simulink model "untitled"  (R2025a)
settings: Solver=VariableStepAuto  StartTime=0.0  StopTime=10.0  RelTol=1e-3
undefined symbols (not defined in the file): b, g, Initial_Point, k, m, mass_0
settings Model: Creator=ACER  LastModifiedBy=ACER

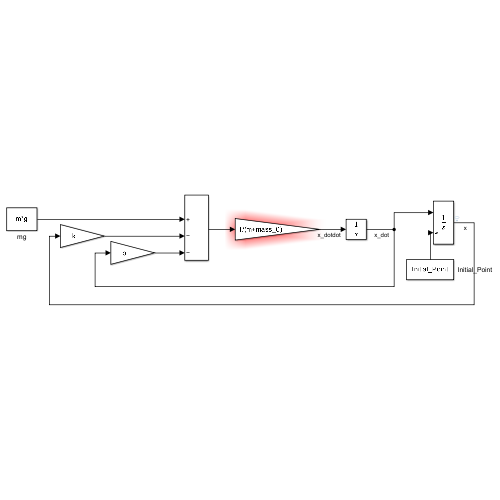
[thumbnail: Simulink's stored preview of the top-level diagram]
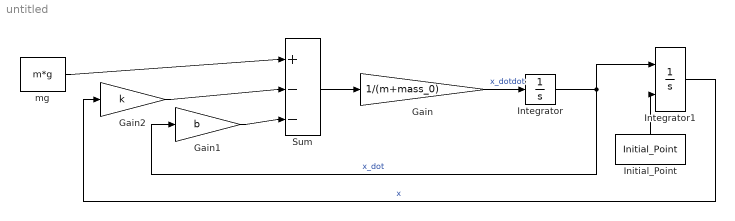
== system untitled ==
  Gain : Gain  Gain=1/(m+mass_0)
  Gain1 : Gain  Gain=b
  Gain2 : Gain  Gain=k
  Initial_Point : Constant  Value=Initial_Point
  Integrator : Integrator
  Integrator1 : Integrator  InitialConditionSource=external
  Sum : Sum  Inputs=|+--
  mg : Constant  Value=m*g
  wires:
  Gain2/1 -> Sum/2
  Gain1/1 -> Sum/3
  mg/1 -> Sum/1
  Sum/1 -> Gain/1
  Integrator/1 -> Gain1/1, Integrator1/1  "x_dot"
  Gain/1 -> Integrator/1  "x_dotdot"
  Integrator1/1 -> Gain2/1  "x"
  Initial_Point/1 -> Integrator1/2
